simulink model "control_sim_ESN_T_only"  (R2022a)
settings: Solver=VariableStepAuto  StartTime=0.0  StopTime=300  RelTol=1e-3
values from neighbouring files (symbols this model uses):
  layersff = {}    [build_ESN.m]    (also in sim_vars2.mat = ; sim_vars_working_temp.mat = )
  layersrcn = {}    [build_ESN.m]    (also in sim_vars2.mat = ; sim_vars_working_temp.mat = )
  tau_nom = 300    [sim_vars2.mat]    (also in sim_vars_working_temp.mat = [300 2.75])
  W_out = [0.0133082466491 -0.0424306072673 0.043897809257 -0.287982408277 0.143010298052 0.163687655935 0.303711686836 0.140929447924 0.227211492369 0.0895156989573 0.103060697293 0.0477229888347 ... (176 elements, 1x176)]    [sim_vars2.mat]    (also in sim_vars_working_temp.mat = [0.0140984265204 -0.0134799639252 -0.00498091522502 0.013951; train_esn.m = y_target*output_series_concat'*((output_series_concat*output)
undefined symbols (not defined in the file or in its folder): normrnd
libraries: dspmtrx3 x2
settings Model: Creator=ripme  LastModifiedBy=ripme

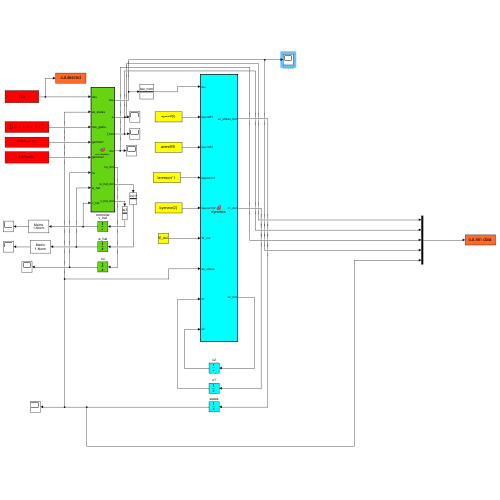
[thumbnail: Simulink's stored preview of the top-level diagram]
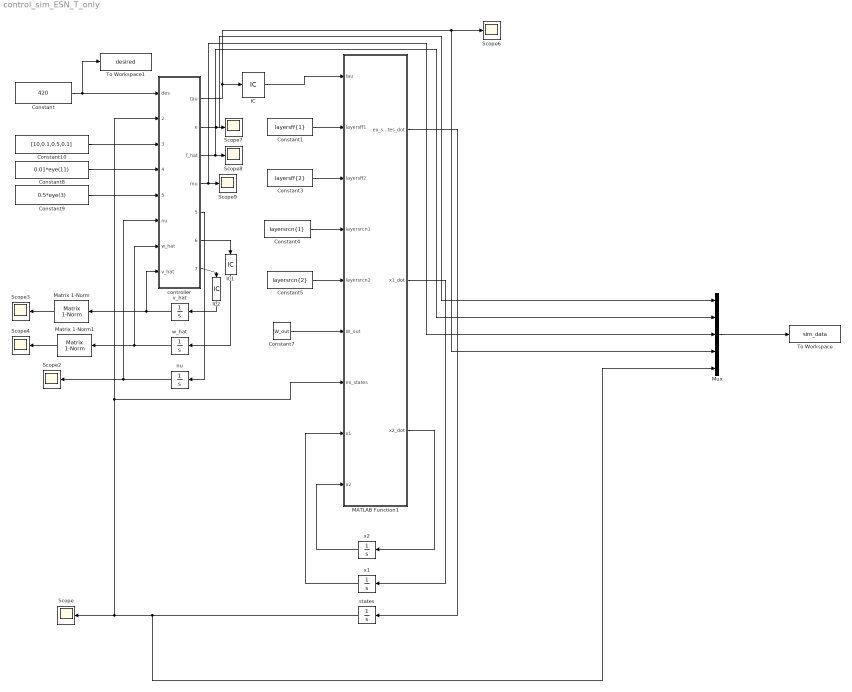
== system control_sim_ESN_T_only ==
  Constant : Constant  Value=420
  Constant1 : Constant  Value=layersff{1}
  Constant10 : Constant  Value=[10,0.1,0.5,0.1]
  Constant3 : Constant  Value=layersff{2}
  Constant4 : Constant  Value=layersrcn{1}
  Constant5 : Constant  Value=layersrcn{2}
  Constant7 : Constant  Value=W_out
  Constant8 : Constant  Value=0.01*eye(11)
  Constant9 : Constant  Value=0.5*eye(3)
  IC : InitialCondition  Value=tau_nom
  IC1 : InitialCondition  Value=zeros(11,1)
  IC2 : InitialCondition  Value=zeros(3,10)
  MATLAB Function1 : MATLAB Function  TreatAsAtomicUnit=on
  Matrix 1-Norm : dspmtrx3/Matrix  1-Norm  roundingMode=Floor  overflowMode=off  outputDataTypeStr=Inherit: Same as accumulator  outputMin=[]  outputMax=[]  outputLastDataTypeStr=Inherit: Same as accumulator
      settings: SourceProductBaseCode=DS
  Matrix 1-Norm1 : dspmtrx3/Matrix  1-Norm  roundingMode=Floor  overflowMode=off  outputDataTypeStr=Inherit: Same as accumulator  outputMin=[]  outputMax=[]  outputLastDataTypeStr=Inherit: Same as accumulator
      settings: SourceProductBaseCode=DS
  Mux : Mux  Inputs=5
  Scope{,2..4,6..9} (8 alike) : Scope
  To Workspace : ToWorkspace  VariableName=sim_data  SampleTime=-1
  To Workspace1 : ToWorkspace  VariableName=desired  SampleTime=-1
  controller : MATLAB Function  TreatAsAtomicUnit=on
  nu : Integrator
  states : Integrator  InitialCondition=410
  v_hat : Integrator  InitialCondition=normrnd(0,0.25,3,10)
  w_hat : Integrator  InitialCondition=zeros(11,1)
  x1 : Integrator  InitialCondition=rand(35,1)
  x2 : Integrator  InitialCondition=rand(88,1)
  wires:
  x1/1 -> MATLAB Function1/8(x1)
  MATLAB Function1/2(x1_dot) -> x1/1
  controller/6(w_hat_dot) -> IC1/1
  v_hat/1 -> controller/8(v_hat), Matrix 1-Norm/1
  w_hat/1 -> controller/7(w_hat), Matrix 1-Norm1/1
  controller/7(v_hat_dot) -> IC2/1
  controller/5(nu_dot) -> nu/1
  nu/1 -> controller/6(nu), Scope2/1
  Constant/1 -> To Workspace1/1, controller/1(des)
  MATLAB Function1/1(ex_states_dot) -> states/1
  MATLAB Function1/3(x2_dot) -> x2/1
  x2/1 -> MATLAB Function1/9(x2)
  states/1 -> Mux/5, Scope/1, controller/2(ex_states), MATLAB Function1/7(ex_states)
  Constant1/1 -> MATLAB Function1/2(layersff1)
  Constant3/1 -> MATLAB Function1/3(layersff2)
  Constant4/1 -> MATLAB Function1/4(layersrcn1)
  Constant5/1 -> MATLAB Function1/5(layersrcn2)
  Constant7/1 -> MATLAB Function1/6(W_out)
  Constant9/1 -> controller/5(gamma2)
  Constant8/1 -> controller/4(gamma1)
  Constant10/1 -> controller/3(rise_gains)
  Matrix 1-Norm/1 -> Scope3/1
  Matrix 1-Norm1/1 -> Scope4/1
  IC/1 -> MATLAB Function1/1(tau)
  IC2/1 -> v_hat/1
  IC1/1 -> w_hat/1
  controller/1(tau) -> Scope6/1, Mux/4, IC/1
  controller/2(e) -> Mux/1, Scope7/1
  controller/3(f_hat) -> Mux/2, Scope8/1
  controller/4(mu) -> Mux/3, Scope9/1
  Mux/1 -> To Workspace/1

== matlab function control_sim_ESN_T_only/MATLAB Function1 ==
  data: tau input; layersff1 input; layersff2 input; layersrcn1 input; layersrcn2 input; W_out input; ex_states_dot output; ex_states input; x1 input; x1_dot output; x2_dot output; x2 input
function [ex_states_dot, x1_dot, x2_dot]= dynamics(tau,layersff1,layersff2,layersrcn1,layersrcn2, W_out, ex_states, x1,x2)

    temp=ex_states;
    omega=tau;
    %{
    temp = temp-420;
    temp = 2*temp/(460-380);
    force = force-550;
    force = 2*force/(700-400);
    %}
    omega = omega-225;
    omega = 2*omega/(400-150);
    input=temp';
    x1_dot = (tanh(layersff1*input)-layersrcn1*x1);
    x2_dot = (tanh(layersff2*x1)-layersrcn2*x2);
    %x3_dot = (tanh(layersff3*x2)-layersrcn3*x3);
    ex_states_dot=W_out'*[tanh(x2);tanh(x2)*omega];
end

== matlab function control_sim_ESN_T_only/controller ==
  data: des input; ex_states input; rise_gains input; gamma1 input; gamma2 input; tau output; e output; f_hat output; mu output; nu input; w_hat input; v_hat input; nu_dot output; w_hat_dot output; v_hat_dot output
function [tau,e,f_hat,mu, nu_dot, w_hat_dot, v_hat_dot] = controller(des,ex_states,rise_gains,gamma1, gamma2, nu, w_hat, v_hat)
    %unpack
    kr = rise_gains(1);
    alpha_r = rise_gains(2);
    gamma_r = rise_gains(3);
    beta_r = rise_gains(4);
    e=des-ex_states;
    e_init=-10;

    tau_nom=300;
    %NN
    xd_vec = [des;ex_states;1]; % (5x1)
    % v (4xL)=(3x5)
    v = v_hat'*xd_vec; % (10x5)(5x1) = (10x1)
    
    %sigma_hat = log(1+exp(v)); % (10x1)
    sigma_hat = 1./(1+exp(-v)); % (10x1)
    
    sigma_vec = [1 sigma_hat']';   % (11x1)

    sigma_prime = sigma_hat.*(1-sigma_hat);
    
    %sigma_prime_vec = [ones(1,10); diag(exp(sigma_hat)./(ones(10,1)+exp(sigma_hat)))]; % (1x10);(10x10)=(11x10)
    sigma_prime_vec = [ones(1,10); diag(sigma_prime)]; % (1x10);(10x10)=(11x10)
    
    f_hat = w_hat'*sigma_vec; % (2x1)
    
    %sigmas(1)*u_h
    w_hat_dot = gamma1*sigma_vec*e'; %(11x11)(11x1)(1x2)=(11x2)
    %w_hat_dot = zeros(11,2); %(11x11)(11x1)(1x2)=(11x2)
    
    v_hat_dot = gamma2*xd_vec*e'*w_hat'*sigma_prime_vec; %(5x5)(5x1)(1x2)(2x11)(11x10)=(5x10)
    %v_hat_dot = zeros(5,10); %(5x5)(5x1)(1x2)(2x11)(11x10)=(5x10)

    %RISE
    mu = kr*e+nu;%kr*e_init+nu;
    %mu(2)=0.01*mu(2);
    nu_dot = (kr*alpha_r+gamma_r)*e+beta_r*sign(e);
    %nu_dot(2)=0.01*nu_dot(2);

    %f_hat(2)=f_hat(2)*0.01;

    tau=tau_nom+mu+f_hat;
    if tau<150 
        tau=150;
        nu_dot=0;
    end
    if tau>450 
        tau=450;
        nu_dot=0;
    end
    %{
    if tau(2)<1 
        tau(2)=1;
    end
    if tau(2)>4 
        tau(2)=1;
    end
    %}
    %tau=[500,4]';
    %tau(2)=2.75;
end
